simulink model "Pipe_simulink (1)"  (R2017b)
settings: Solver=VariableStepAuto  StartTime=0.0  StopTime=10.0  RelTol=1e-3
settings Model: Creator=Siddharth  LastModifiedBy=Siddharth

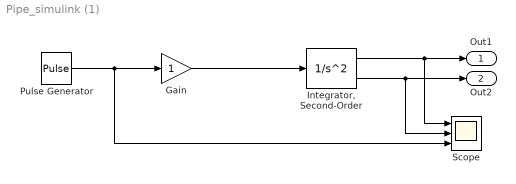
== system Pipe_simulink (1) ==
  Gain : Gain
  "Integrator, Second-Order" : SecondOrderIntegrator
  Pulse Generator : DiscretePulseGenerator  PulseType=Time based  Period=1  PulseWidth=50
  Scope : Scope  NumInputPorts=3
  Out1 : Outport
  Out2 : Outport  Port=2
  wires:
  Pulse Generator/1 -> Scope/3, Gain/1
  Gain/1 -> "Integrator, Second-Order"/1
  "Integrator, Second-Order"/1 -> Scope/1, Out1/1
  "Integrator, Second-Order"/2 -> Scope/2, Out2/1
